simulink model "CMOS_Kernel_Memory_Sync"  (R2023b)
settings: Solver=VariableStepAuto  StartTime=0.0  StopTime=30000000  RelTol=1e-3
values from neighbouring files (symbols this model uses):
  AmountOfPixelsPerScanline = 400    [Kernel_Setup_Script.m]
  AmountOfRamBlocksScanlines = 5    [Kernel_Setup_Script.m]
  AmountOfRamBlocksScanlinesOffset = AmountOfRamBlocksScanlines - 1    (= 4)    [Kernel_Setup_Script.m]
  AmountOfScanlinePixels = 73700    [Kernel_Setup_Script.m]
  AmountOfScanlinePixelsOffset = AmountOfScanlinePixels - 1    (= 73699)    [Kernel_Setup_Script.m]
  AmountOfScanlines = 1100    [Kernel_Setup_Script.m]
  AmountOfScanlinesOffset = AmountOfScanlines - 1    (= 1099)    [Kernel_Setup_Script.m]
  AOPPK_Off = AmountOfPixelsPerScanline - 1    (= 399)    [Kernel_Setup_Script.m]
  AOPPS_Off = AmountOfPixelsPerScanline - 1    (= 399)    [Kernel_Setup_Script.m]
  FramePackOff_0 = FramePackOff_0 - ScanlineFifoCheck    [Kernel_Setup_Script.m]
  FramePackOff_1 = FramePackOff_1 - ScanlineFifoCheck    [Kernel_Setup_Script.m]
  FramePackOff_2 = FramePackOff_2 - ScanlineFifoCheck    [Kernel_Setup_Script.m]
  FramePackOff_3 = FramePackOff_3 - ScanlineFifoCheck    [Kernel_Setup_Script.m]
  FramePackOff_4 = FramePackOff_4 - ScanlineFifoCheck    [Kernel_Setup_Script.m]
  FramePackOff_5 = FramePackOff_5 - ScanlineFifoCheck    [Kernel_Setup_Script.m]
  KernelPackOff_0 = KernelPackOff_0 - KernelBitsPerRow    [Kernel_Setup_Script.m]
  KernelPackOff_1 = KernelPackOff_1 - KernelBitsPerRow    [Kernel_Setup_Script.m]
  KernelPackOff_2 = KernelPackOff_2 - KernelBitsPerRow    [Kernel_Setup_Script.m]
  KernelPackOff_3 = KernelPackOff_3 - KernelBitsPerRow    [Kernel_Setup_Script.m]
  Slice59DownTo48Top = (MsbOffset - (ScanlinePixelBitSizeController*1))    (= 59)    [Kernel_Setup_Script.m]
  Slice71DownTo60Top = (MsbOffset - (ScanlinePixelBitSizeController*0))    (= 71)    [Kernel_Setup_Script.m]
  TotalSectionsForFrames = AmountOfScanlines/AmountOfRamBlocksScanlines    (= 220)    [Kernel_Setup_Script.m]
  UltraRamRows = AmountOfPixelsPerScanline/ScanlineFifoCheck    [Kernel_Setup_Script.m]
  UltraRamRowsCeil = ceil(AmountOfPixelsPerScanline/ScanlineFifoCheck)    [Kernel_Setup_Script.m]
  UltraRamRowsKernel = AmountOfPixelsPerScanline/KernelBitsPerRow    (= 100)    [Kernel_Setup_Script.m]
  UltraRamRowsKernelCeil = ceil(AmountOfPixelsPerScanline/KernelBitsPerRow)    [Kernel_Setup_Script.m]
  UltraRamRowsMemorySectionOffset = UltraRamRowsCeil*AmountOfRamBlocksScanlines    [Kernel_Setup_Script.m]
  UltraRamRowsOffset = UltraRamRowsCeil - 1    [Kernel_Setup_Script.m]
undefined symbols (not defined in the file or in its folder): c, Down, sfvc784, Up, xck26
libraries: hdlBasic x4512, vmcUtilities x1
(part 2 of 39)

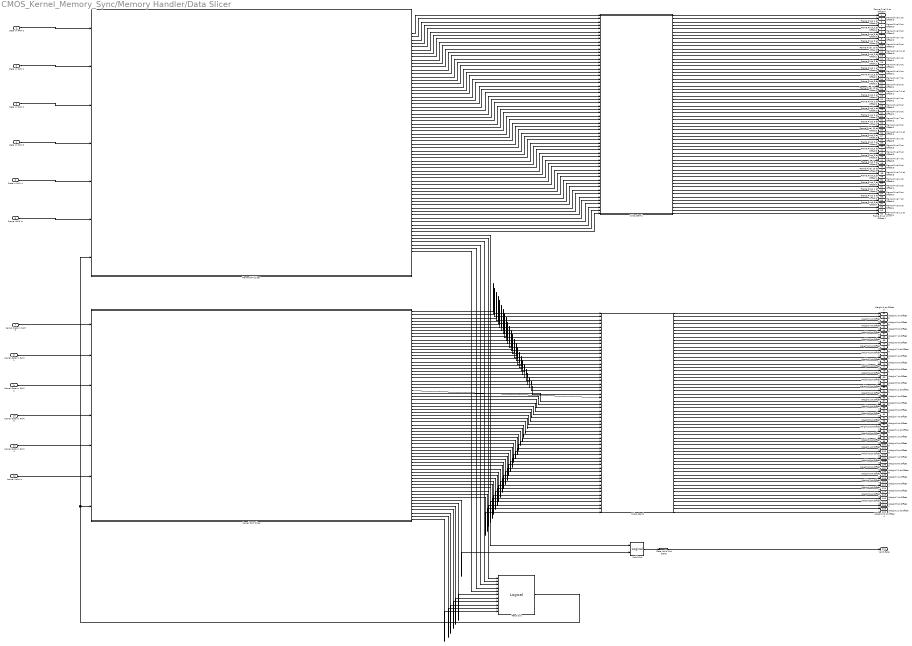
== system CMOS_Kernel_Memory_Sync/Memory Handler/Data Slicer ==
  Data In RAM 0 : Inport
  Data In RAM 1 : Inport  Port=2
  Data In RAM 2 : Inport  Port=3
  Data In RAM 3 : Inport  Port=4
  Data In RAM 4 : Inport  Port=5
  Frame Valid In : Inport  Port=6
  Kernel Data In RAM 0 : Inport  Port=7
  Kernel Data In RAM 1 : Inport  Port=8
  Kernel Data In RAM 2 : Inport  Port=9
  Kernel Data In RAM 3 : Inport  Port=10
  Kernel Data In RAM 4 : Inport  Port=11
  Kernel Valid In : Inport  Port=12
  Data Valid Out Delay : hdlBasic/Delay  rst=off  en=off  latency=1  reg_retiming=off  XmcBlockStatus=1  maskContainerNames=group1  block_type=delay  block_config=sysgen:Delay_config
  Frame RAM Slicer : Subsystem
      settings: RTWMemSecFuncInitTerm=Inherit fRAM model  RTWMemSecFuncExecute=Inherit fRAM model  RTWMemSecDataConstants=Inherit fRAM model  RTWMemSecDataInternal=Inherit fRAM model  RTWMemSecDataParameters=Inherit fRAM model
  Kernel RAM Slicer : Subsystem
      settings: RTWMemSecFuncInitTerm=Inherit fRAM model  RTWMemSecFuncExecute=Inherit fRAM model  RTWMemSecDataConstants=Inherit fRAM model  RTWMemSecDataInternal=Inherit fRAM model  RTWMemSecDataParameters=Inherit fRAM model
  Read Out : hdlBasic/Logical  logical_function=AND  inputs=11  en=off  latency=1  precision=User Defined  arith_type=Boolean  n_bits=1  bin_pt=0  align_bp=on  overflow=[]  quantization=[]  XmcBlockStatus=1  maskContainerNames=tabcontainer1  block_type=logical  block_config=sysgen:Logical_config
  Subsystem1 : Subsystem
      settings: RTWMemSecFuncInitTerm=Inherit fRAM model  RTWMemSecFuncExecute=Inherit fRAM model  RTWMemSecDataConstants=Inherit fRAM model  RTWMemSecDataInternal=Inherit fRAM model  RTWMemSecDataParameters=Inherit fRAM model
  Subsystem2 : Subsystem
      settings: RTWMemSecFuncInitTerm=Inherit fRAM model  RTWMemSecFuncExecute=Inherit fRAM model  RTWMemSecDataConstants=Inherit fRAM model  RTWMemSecDataInternal=Inherit fRAM model  RTWMemSecDataParameters=Inherit fRAM model
  Valid Out : hdlBasic/Logical  logical_function=AND  inputs=2  en=off  latency=1  precision=Full  arith_type=Unsigned  n_bits=16  bin_pt=0  align_bp=on  overflow=[]  quantization=[]  XmcBlockStatus=1  maskContainerNames=tabcontainer1  block_type=logical  block_config=sysgen:Logical_config
  Frame Pixel 0 at Offset 0 : Outport
  Frame Pixel 1 at Offset 0 : Outport  Port=2
  Frame Pixel 2 at Offset 0 : Outport  Port=3
  Frame Pixel 3 at Offset 0 : Outport  Port=4
  Frame Pixel 4 at Offset 0 : Outport  Port=5
  Frame Pixel 5 at Offset 0 : Outport  Port=6
  Frame Pixel 6 at Offset 0 : Outport  Port=7
  Frame Pixel 7 at Offset 0 : Outport  Port=8
  Frame Pixel 8 at Offset 0 : Outport  Port=9
  Frame Pixel 9 at Offset 0 : Outport  Port=10
  Frame Pixel 10 at Offset 0 : Outport  Port=11
  Frame Pixel 11 at Offset 0 : Outport  Port=12
  Frame Pixel 0 at Offset 1 : Outport  Port=13
  Frame Pixel 1 at Offset 1 : Outport  Port=14
  Frame Pixel 2 at Offset 1 : Outport  Port=15
  Frame Pixel 3 at Offset 1 : Outport  Port=16
  Frame Pixel 4 at Offset 1 : Outport  Port=17
  Frame Pixel 5 at Offset 1 : Outport  Port=18
  Frame Pixel 6 at Offset 1 : Outport  Port=19
  Frame Pixel 7 at Offset 1 : Outport  Port=20
  Frame Pixel 8 at Offset 1 : Outport  Port=21
  Frame Pixel 9 at Offset 1 : Outport  Port=22
  Frame Pixel 10 at Offset 1 : Outport  Port=23
  Frame Pixel 11 at Offset 1 : Outport  Port=24
  Frame Pixel 0 at Offset 2 : Outport  Port=25
  Frame Pixel 1 at Offset 2 : Outport  Port=26
  Frame Pixel 2 at Offset 2 : Outport  Port=27
  Frame Pixel 3 at Offset 2 : Outport  Port=28
  Frame Pixel 4 at Offset 2 : Outport  Port=29
  Frame Pixel 5 at Offset 2 : Outport  Port=30
  Frame Pixel 6 at Offset 2 : Outport  Port=31
  Frame Pixel 7 at Offset 2 : Outport  Port=32
  Frame Pixel 8 at Offset 2 : Outport  Port=33
  Frame Pixel 9 at Offset 2 : Outport  Port=34
  Frame Pixel 10 at Offset 2 : Outport  Port=35
  Frame Pixel 11 at Offset 2 : Outport  Port=36
  Frame Pixel 0 at Offset 3 : Outport  Port=37
  Frame Pixel 1 at Offset 3 : Outport  Port=38
  Frame Pixel 2 at Offset 3 : Outport  Port=39
  Frame Pixel 3 at Offset 3 : Outport  Port=40
  Frame Pixel 4 at Offset 3 : Outport  Port=41
  Frame Pixel 5 at Offset 3 : Outport  Port=42
  Frame Pixel 6 at Offset 3 : Outport  Port=43
  Frame Pixel 7 at Offset 3 : Outport  Port=44
  Frame Pixel 8 at Offset 3 : Outport  Port=45
  Frame Pixel 9 at Offset 3 : Outport  Port=46
  Frame Pixel 10 at Offset 3 : Outport  Port=47
  Frame Pixel 11 at Offset 3 : Outport  Port=48
  Frame Pixel 0 at Offset 4 : Outport  Port=49
  Frame Pixel 1 at Offset 4 : Outport  Port=50
  Frame Pixel 2 at Offset 4 : Outport  Port=51
  Frame Pixel 3 at Offset 4 : Outport  Port=52
  Frame Pixel 4 at Offset 4 : Outport  Port=53
  Frame Pixel 5 at Offset 4 : Outport  Port=54
  Frame Pixel 6 at Offset 4 : Outport  Port=55
  Frame Pixel 7 at Offset 4 : Outport  Port=56
  Frame Pixel 8 at Offset 4 : Outport  Port=57
  Frame Pixel 9 at Offset 4 : Outport  Port=58
  Frame Pixel 10 at Offset 4 : Outport  Port=59
  Frame Pixel 11 at Offset 4 : Outport  Port=60
  Weight 0 at Offset 0 : Outport  Port=61
  Weight 1 at Offset 0 : Outport  Port=62
  Weight 2 at Offset 0 : Outport  Port=63
  Weight 3 at Offset 0 : Outport  Port=64
  Weight 4 at Offset 0 : Outport  Port=65
  Weight 5 at Offset 0 : Outport  Port=66
  Weight 6 at Offset 0 : Outport  Port=67
  Weight 7 at Offset 0 : Outport  Port=68
  Weight 8 at Offset 0 : Outport  Port=69
  Weight 9 at Offset 0 : Outport  Port=70
  Weight 10 at Offset 0 : Outport  Port=71
  Weight 11 at Offset 0 : Outport  Port=72
  Weight 0 at Offset 1 : Outport  Port=73
  Weight 1 at Offset 1 : Outport  Port=74
  Weight 2 at Offset 1 : Outport  Port=75
  Weight 3 at Offset 1 : Outport  Port=76
  Weight 4 at Offset 1 : Outport  Port=77
  Weight 5 at Offset 1 : Outport  Port=78
  Weight 6 at Offset 1 : Outport  Port=79
  Weight 7 at Offset 1 : Outport  Port=80
  Weight 8 at Offset 1 : Outport  Port=81
  Weight 9 at Offset 1 : Outport  Port=82
  Weight 10 at Offset 1 : Outport  Port=83
  Weight 11 at Offset 1 : Outport  Port=84
  Weight 0 at Offset 2 : Outport  Port=85
  Weight 1 at Offset 2 : Outport  Port=86
  Weight 2 at Offset 2 : Outport  Port=87
  Weight 3 at Offset 2 : Outport  Port=88
  Weight 4 at Offset 2 : Outport  Port=89
  Weight 5 at Offset 2 : Outport  Port=90
  Weight 6 at Offset 2 : Outport  Port=91
  Weight 7 at Offset 2 : Outport  Port=92
  Weight 8 at Offset 2 : Outport  Port=93
  Weight 9 at Offset 2 : Outport  Port=94
  Weight 10 at Offset 2 : Outport  Port=95
  Weight 11 at Offset 2 : Outport  Port=96
  Weight 0 at Offset 3 : Outport  Port=97
  Weight 1 at Offset 3 : Outport  Port=98
  Weight 2 at Offset 3 : Outport  Port=99
  Weight 3 at Offset 3 : Outport  Port=100
  Weight 4 at Offset 3 : Outport  Port=101
  Weight 5 at Offset 3 : Outport  Port=102
  Weight 6 at Offset 3 : Outport  Port=103
  Weight 7 at Offset 3 : Outport  Port=104
  Weight 8 at Offset 3 : Outport  Port=105
  Weight 9 at Offset 3 : Outport  Port=106
  Weight 10 at Offset 3 : Outport  Port=107
  Weight 11 at Offset 3 : Outport  Port=108
  Weight 0 at Offset 4 : Outport  Port=109
  Weight 1 at Offset 4 : Outport  Port=110
  Weight 2 at Offset 4 : Outport  Port=111
  Weight 3 at Offset 4 : Outport  Port=112
  Weight 4 at Offset 4 : Outport  Port=113
  Weight 5 at Offset 4 : Outport  Port=114
  Weight 6 at Offset 4 : Outport  Port=115
  Weight 7 at Offset 4 : Outport  Port=116
  Weight 8 at Offset 4 : Outport  Port=117
  Weight 9 at Offset 4 : Outport  Port=118
  Weight 10 at Offset 4 : Outport  Port=119
  Weight 11 at Offset 4 : Outport  Port=120
  Valid Data : Outport  Port=121
  wires:
  Kernel RAM Slicer/61(Valid Out) -> Valid Out/2
  Frame RAM Slicer/61(Valid Out) -> Valid Out/1
  Frame RAM Slicer/1(Frame 12 Bit Bin Value 0 RAM 0) -> Subsystem1/1(Frame 12 Bit Bin Value 0)
  Frame RAM Slicer/2(Frame 12 Bit Bin Value 1 RAM 0) -> Subsystem1/2(Frame 12 Bit Bin Value 1)
  Frame RAM Slicer/3(Frame 12 Bit Bin Value 2 RAM 0) -> Subsystem1/3(Frame 12 Bit Bin Value 2)
  Frame RAM Slicer/4(Frame 12 Bit Bin Value 3 RAM 0) -> Subsystem1/4(Frame 12 Bit Bin Value 3)
  Frame RAM Slicer/5(Frame 12 Bit Bin Value 4 RAM 0) -> Subsystem1/5(Frame 12 Bit Bin Value 4)
  Frame RAM Slicer/6(Frame 12 Bit Bin Value 5 RAM 0) -> Subsystem1/6(Frame 12 Bit Bin Value 5)
  Frame RAM Slicer/7(Frame 12 Bit Bin Value 6 RAM 0) -> Subsystem1/7(Frame 12 Bit Bin Value 6)
  Frame RAM Slicer/8(Frame 12 Bit Bin Value 7 RAM 0) -> Subsystem1/8(Frame 12 Bit Bin Value 7)
  Frame RAM Slicer/9(Frame 12 Bit Bin Value 8 RAM 0) -> Subsystem1/9(Frame 12 Bit Bin Value 8)
  Frame RAM Slicer/10(Frame 12 Bit Bin Value 9 RAM 0) -> Subsystem1/10(Frame 12 Bit Bin Value 9)
  Frame RAM Slicer/11(Frame 12 Bit Bin Value 10 RAM 0) -> Subsystem1/11(Frame 12 Bit Bin Value 10)
  Frame RAM Slicer/12(Frame 12 Bit Bin Value 11 RAM 0) -> Subsystem1/12(Frame 12 Bit Bin Value 11)
  Frame RAM Slicer/13(Frame 12 Bit Bin Value 0 RAM 1) -> Subsystem1/13(Frame 12 Bit Bin Value 12)
  Frame RAM Slicer/14(Frame 12 Bit Bin Value 1 RAM 1) -> Subsystem1/14(Frame 12 Bit Bin Value 13)
  Frame RAM Slicer/15(Frame 12 Bit Bin Value 2 RAM 1) -> Subsystem1/15(Frame 12 Bit Bin Value 14)
  Frame RAM Slicer/16(Frame 12 Bit Bin Value 3 RAM 1) -> Subsystem1/16(Frame 12 Bit Bin Value 15)
  Frame RAM Slicer/17(Frame 12 Bit Bin Value 4 RAM 1) -> Subsystem1/17(Frame 12 Bit Bin Value 16)
  Frame RAM Slicer/18(Frame 12 Bit Bin Value 5 RAM 1) -> Subsystem1/18(Frame 12 Bit Bin Value 17)
  Frame RAM Slicer/19(Frame 12 Bit Bin Value 6 RAM 1) -> Subsystem1/19(Frame 12 Bit Bin Value 18)
  Frame RAM Slicer/20(Frame 12 Bit Bin Value 7 RAM 1) -> Subsystem1/20(Frame 12 Bit Bin Value 19)
  Frame RAM Slicer/21(Frame 12 Bit Bin Value 8 RAM 1) -> Subsystem1/21(Frame 12 Bit Bin Value 20)
  Frame RAM Slicer/22(Frame 12 Bit Bin Value 9 RAM 1) -> Subsystem1/22(Frame 12 Bit Bin Value 21)
  Frame RAM Slicer/23(Frame 12 Bit Bin Value 10 RAM 1) -> Subsystem1/23(Frame 12 Bit Bin Value 22)
  Frame RAM Slicer/24(Frame 12 Bit Bin Value 11 RAM 1) -> Subsystem1/24(Frame 12 Bit Bin Value 23)
  Frame RAM Slicer/25(Frame 12 Bit Bin Value 0 RAM 2) -> Subsystem1/25(Frame 12 Bit Bin Value 24)
  Frame RAM Slicer/26(Frame 12 Bit Bin Value 1 RAM 2) -> Subsystem1/26(Frame 12 Bit Bin Value 25)
  Frame RAM Slicer/27(Frame 12 Bit Bin Value 2 RAM 2) -> Subsystem1/27(Frame 12 Bit Bin Value 26)
  Frame RAM Slicer/28(Frame 12 Bit Bin Value 3 RAM 2) -> Subsystem1/28(Frame 12 Bit Bin Value 27)
  Frame RAM Slicer/29(Frame 12 Bit Bin Value 4 RAM 2) -> Subsystem1/29(Frame 12 Bit Bin Value 28)
  Frame RAM Slicer/30(Frame 12 Bit Bin Value 5 RAM 2) -> Subsystem1/30(Frame 12 Bit Bin Value 29)
  Frame RAM Slicer/31(Frame 12 Bit Bin Value 6 RAM 2) -> Subsystem1/31(Frame 12 Bit Bin Value 30)
  Frame RAM Slicer/32(Frame 12 Bit Bin Value 7 RAM 2) -> Subsystem1/32(Frame 12 Bit Bin Value 31)
  Frame RAM Slicer/33(Frame 12 Bit Bin Value 8 RAM 2) -> Subsystem1/33(Frame 12 Bit Bin Value 32)
  Frame RAM Slicer/34(Frame 12 Bit Bin Value 9 RAM 2) -> Subsystem1/34(Frame 12 Bit Bin Value 33)
  Frame RAM Slicer/35(Frame 12 Bit Bin Value 10 RAM 2) -> Subsystem1/35(Frame 12 Bit Bin Value 34)
  Frame RAM Slicer/36(Frame 12 Bit Bin Value 11 RAM 2) -> Subsystem1/36(Frame 12 Bit Bin Value 35)
  Frame RAM Slicer/42(Frame 12 Bit Bin Value 5 RAM 3) -> Subsystem1/42(Frame 12 Bit Bin Value 41)
  Frame RAM Slicer/37(Frame 12 Bit Bin Value 0 RAM 3) -> Subsystem1/37(Frame 12 Bit Bin Value 36)
  Frame RAM Slicer/54(Frame 12 Bit Bin Value 5 RAM 4) -> Subsystem1/54(Frame 12 Bit Bin Value 53)
  Frame RAM Slicer/57(Frame 12 Bit Bin Value 8 RAM 4) -> Subsystem1/57(Frame 12 Bit Bin Value 56)
  Frame RAM Slicer/47(Frame 12 Bit Bin Value 10 RAM 3) -> Subsystem1/47(Frame 12 Bit Bin Value 46)
  Frame RAM Slicer/53(Frame 12 Bit Bin Value 4 RAM 4) -> Subsystem1/53(Frame 12 Bit Bin Value 52)
  Frame RAM Slicer/44(Frame 12 Bit Bin Value 7 RAM 3) -> Subsystem1/44(Frame 12 Bit Bin Value 43)
  Frame RAM Slicer/51(Frame 12 Bit Bin Value 2 RAM 4) -> Subsystem1/51(Frame 12 Bit Bin Value 50)
  Frame RAM Slicer/58(Frame 12 Bit Bin Value 9 RAM 4) -> Subsystem1/58(Frame 12 Bit Bin Value 57)
  Frame RAM Slicer/56(Frame 12 Bit Bin Value 7 RAM 4) -> Subsystem1/56(Frame 12 Bit Bin Value 55)
  Frame RAM Slicer/52(Frame 12 Bit Bin Value 3 RAM 4) -> Subsystem1/52(Frame 12 Bit Bin Value 51)
  Frame RAM Slicer/43(Frame 12 Bit Bin Value 6 RAM 3) -> Subsystem1/43(Frame 12 Bit Bin Value 42)
  Frame RAM Slicer/49(Frame 12 Bit Bin Value 0 RAM 4) -> Subsystem1/49(Frame 12 Bit Bin Value 48)
  Frame RAM Slicer/40(Frame 12 Bit Bin Value 3 RAM 3) -> Subsystem1/40(Frame 12 Bit Bin Value 39)
  Frame RAM Slicer/46(Frame 12 Bit Bin Value 9 RAM 3) -> Subsystem1/46(Frame 12 Bit Bin Value 45)
  Frame RAM Slicer/55(Frame 12 Bit Bin Value 6 RAM 4) -> Subsystem1/55(Frame 12 Bit Bin Value 54)
  Frame RAM Slicer/39(Frame 12 Bit Bin Value 2 RAM 3) -> Subsystem1/39(Frame 12 Bit Bin Value 38)
  Frame RAM Slicer/45(Frame 12 Bit Bin Value 8 RAM 3) -> Subsystem1/45(Frame 12 Bit Bin Value 44)
  Frame RAM Slicer/60(Frame 12 Bit Bin Value 11 RAM 4) -> Subsystem1/60(Frame 12 Bit Bin Value 59)
  Frame RAM Slicer/59(Frame 12 Bit Bin Value 10 RAM 4) -> Subsystem1/59(Frame 12 Bit Bin Value 58)
  Frame RAM Slicer/41(Frame 12 Bit Bin Value 4 RAM 3) -> Subsystem1/41(Frame 12 Bit Bin Value 40)
  Frame RAM Slicer/50(Frame 12 Bit Bin Value 1 RAM 4) -> Subsystem1/50(Frame 12 Bit Bin Value 49)
  Frame RAM Slicer/48(Frame 12 Bit Bin Value 11 RAM 3) -> Subsystem1/48(Frame 12 Bit Bin Value 47)
  Frame RAM Slicer/38(Frame 12 Bit Bin Value 1 RAM 3) -> Subsystem1/38(Frame 12 Bit Bin Value 37)
  Data In RAM 0/1 -> Frame RAM Slicer/1(Data In RAM 0)
  Data In RAM 2/1 -> Frame RAM Slicer/3(Data In RAM 2)
  Data In RAM 3/1 -> Frame RAM Slicer/4(Data In RAM 3)
  Data In RAM 4/1 -> Frame RAM Slicer/5(Data In RAM 4)
  Frame Valid In/1 -> Frame RAM Slicer/6(Valid In)
  Kernel Data In RAM 0/1 -> Kernel RAM Slicer/1(Kernel Data In RAM 0)
  Kernel Data In RAM 1/1 -> Kernel RAM Slicer/2(Kernel Data In RAM 1)
  Kernel Data In RAM 2/1 -> Kernel RAM Slicer/3(Kernel Data In RAM 2)
  Kernel Data In RAM 3/1 -> Kernel RAM Slicer/4(Kernel Data In RAM 3)
  Kernel Data In RAM 4/1 -> Kernel RAM Slicer/5(Kernel Data In RAM 4)
  Kernel Valid In/1 -> Kernel RAM Slicer/6(Valid In)
  Data In RAM 1/1 -> Frame RAM Slicer/2(Data In RAM 1)
  Valid Out/1 -> Data Valid Out Delay/1
  Kernel RAM Slicer/1(Kernel 18 Bit Value 0 RAM 0) -> Subsystem2/1(Kernel 18 Bit Bin Value 0)
  Kernel RAM Slicer/2(Kernel 18 Bit Value 1 RAM 0) -> Subsystem2/2(Kernel 18 Bit Bin Value 1)
  Kernel RAM Slicer/3(Kernel 18 Bit Value 2 RAM 0) -> Subsystem2/3(Kernel 18 Bit Bin Value 2)
  Kernel RAM Slicer/4(Kernel 18 Bit Value 3 RAM 0) -> Subsystem2/4(Kernel 18 Bit Bin Value 3)
  Kernel RAM Slicer/5(Kernel 18 Bit Value 4 RAM 0) -> Subsystem2/5(Kernel 18 Bit Bin Value 4)
  Kernel RAM Slicer/6(Kernel 18 Bit Value 5 RAM 0) -> Subsystem2/6(Kernel 18 Bit Bin Value 5)
  Kernel RAM Slicer/7(Kernel 18 Bit Value 6 RAM 0) -> Subsystem2/7(Kernel 18 Bit Bin Value 6)
  Kernel RAM Slicer/8(Kernel 18 Bit Value 7 RAM 0) -> Subsystem2/8(Kernel 18 Bit Bin Value 7)
  Kernel RAM Slicer/9(Kernel 18 Bit Value 8 RAM 0) -> Subsystem2/9(Kernel 18 Bit Bin Value 8)
  Kernel RAM Slicer/10(Kernel 18 Bit Value 9 RAM 0) -> Subsystem2/10(Kernel 18 Bit Bin Value 9)
  Kernel RAM Slicer/11(Kernel 18 Bit Value 10 RAM 0) -> Subsystem2/11(Kernel 18 Bit Bin Value 10)
  Kernel RAM Slicer/12(Kernel 18 Bit Value 11 RAM 0) -> Subsystem2/12(Kernel 18 Bit Bin Value 11)
  Kernel RAM Slicer/13(Kernel 18 Bit Value 0 RAM 1) -> Subsystem2/13(Kernel 18 Bit Bin Value 12)
  Kernel RAM Slicer/14(Kernel 18 Bit Value 1 RAM 1) -> Subsystem2/14(Kernel 18 Bit Bin Value 13)
  Kernel RAM Slicer/15(Kernel 18 Bit Value 2 RAM 1) -> Subsystem2/15(Kernel 18 Bit Bin Value 14)
  Kernel RAM Slicer/16(Kernel 18 Bit Value 3 RAM 1) -> Subsystem2/16(Kernel 18 Bit Bin Value 15)
  Kernel RAM Slicer/17(Kernel 18 Bit Value 4 RAM 1) -> Subsystem2/17(Kernel 18 Bit Bin Value 16)
  Kernel RAM Slicer/18(Kernel 18 Bit Value 5 RAM 1) -> Subsystem2/18(Kernel 18 Bit Bin Value 17)
  Kernel RAM Slicer/19(Kernel 18 Bit Value 6 RAM 1) -> Subsystem2/19(Kernel 18 Bit Bin Value 18)
  Kernel RAM Slicer/20(Kernel 18 Bit Value 7 RAM 1) -> Subsystem2/20(Kernel 18 Bit Bin Value 19)
  Kernel RAM Slicer/21(Kernel 18 Bit Value 8 RAM 1) -> Subsystem2/21(Kernel 18 Bit Bin Value 20)
  Kernel RAM Slicer/22(Kernel 18 Bit Value 9 RAM 1) -> Subsystem2/22(Kernel 18 Bit Bin Value 21)
  Kernel RAM Slicer/23(Kernel 18 Bit Value 10 RAM 1) -> Subsystem2/23(Kernel 18 Bit Bin Value 22)
  Kernel RAM Slicer/24(Kernel 18 Bit Value 11 RAM 1) -> Subsystem2/24(Kernel 18 Bit Bin Value 23)
  Kernel RAM Slicer/25(Kernel 18 Bit Value 0 RAM 2) -> Subsystem2/25(Kernel 18 Bit Bin Value 24)
  Kernel RAM Slicer/26(Kernel 18 Bit Value 1 RAM 2) -> Subsystem2/26(Kernel 18 Bit Bin Value 25)
  Kernel RAM Slicer/27(Kernel 18 Bit Value 2 RAM 2) -> Subsystem2/27(Kernel 18 Bit Bin Value 26)
  Kernel RAM Slicer/28(Kernel 18 Bit Value 3 RAM 2) -> Subsystem2/28(Kernel 18 Bit Bin Value 27)
  Kernel RAM Slicer/29(Kernel 18 Bit Value 4 RAM 2) -> Subsystem2/29(Kernel 18 Bit Bin Value 28)
  Kernel RAM Slicer/30(Kernel 18 Bit Value 5 RAM 2) -> Subsystem2/30(Kernel 18 Bit Bin Value 29)
  Kernel RAM Slicer/31(Kernel 18 Bit Value 6 RAM 2) -> Subsystem2/31(Kernel 18 Bit Bin Value 30)
  Kernel RAM Slicer/32(Kernel 18 Bit Value 7 RAM 2) -> Subsystem2/32(Kernel 18 Bit Bin Value 31)
  Kernel RAM Slicer/33(Kernel 18 Bit Value 8 RAM 2) -> Subsystem2/33(Kernel 18 Bit Bin Value 32)
  Kernel RAM Slicer/34(Kernel 18 Bit Value 9 RAM 2) -> Subsystem2/34(Kernel 18 Bit Bin Value 33)
  Kernel RAM Slicer/35(Kernel 18 Bit Value 10 RAM 2) -> Subsystem2/35(Kernel 18 Bit Bin Value 34)
  Kernel RAM Slicer/36(Kernel 18 Bit Value 11 RAM 2) -> Subsystem2/36(Kernel 18 Bit Bin Value 35)
  Kernel RAM Slicer/37(Kernel 18 Bit Value 0 RAM 3) -> Subsystem2/37(Kernel 18 Bit Bin Value 36)
  Kernel RAM Slicer/38(Kernel 18 Bit Value 1 RAM 3) -> Subsystem2/38(Kernel 18 Bit Bin Value 37)
  Kernel RAM Slicer/39(Kernel 18 Bit Value 2 RAM 3) -> Subsystem2/39(Kernel 18 Bit Bin Value 38)
  Kernel RAM Slicer/40(Kernel 18 Bit Value 3 RAM 3) -> Subsystem2/40(Kernel 18 Bit Bin Value 39)
  Kernel RAM Slicer/41(Kernel 18 Bit Value 4 RAM 3) -> Subsystem2/41(Kernel 18 Bit Bin Value 40)
  Kernel RAM Slicer/42(Kernel 18 Bit Value 5 RAM 3) -> Subsystem2/42(Kernel 18 Bit Bin Value 41)
  Kernel RAM Slicer/43(Kernel 18 Bit Value 6 RAM 3) -> Subsystem2/43(Kernel 18 Bit Bin Value 42)
  Kernel RAM Slicer/44(Kernel 18 Bit Value 7 RAM 3) -> Subsystem2/44(Kernel 18 Bit Bin Value 43)
  Kernel RAM Slicer/45(Kernel 18 Bit Value 8 RAM 3) -> Subsystem2/45(Kernel 18 Bit Bin Value 44)
  Kernel RAM Slicer/46(Kernel 18 Bit Value 9 RAM 3) -> Subsystem2/46(Kernel 18 Bit Bin Value 45)
  Kernel RAM Slicer/47(Kernel 18 Bit Value 10 RAM 3) -> Subsystem2/47(Kernel 18 Bit Bin Value 46)
  Kernel RAM Slicer/48(Kernel 18 Bit Value 11 RAM 3) -> Subsystem2/48(Kernel 18 Bit Bin Value 47)
  Kernel RAM Slicer/49(Kernel 18 Bit Value 0 RAM 4) -> Subsystem2/49(Kernel 18 Bit Bin Value 48)
  Kernel RAM Slicer/50(Kernel 18 Bit Value 1 RAM 4) -> Subsystem2/50(Kernel 18 Bit Bin Value 49)
  Kernel RAM Slicer/51(Kernel 18 Bit Value 2 RAM 4) -> Subsystem2/51(Kernel 18 Bit Bin Value 50)
  Kernel RAM Slicer/52(Kernel 18 Bit Value 3 RAM 4) -> Subsystem2/52(Kernel 18 Bit Bin Value 51)
  Kernel RAM Slicer/53(Kernel 18 Bit Value 4 RAM 4) -> Subsystem2/53(Kernel 18 Bit Bin Value 52)
  Kernel RAM Slicer/54(Kernel 18 Bit Value 5 RAM 4) -> Subsystem2/54(Kernel 18 Bit Bin Value 53)
  Kernel RAM Slicer/55(Kernel 18 Bit Value 6 RAM 4) -> Subsystem2/55(Kernel 18 Bit Bin Value 54)
  Kernel RAM Slicer/56(Kernel 18 Bit Value 7 RAM 4) -> Subsystem2/56(Kernel 18 Bit Bin Value 55)
  Kernel RAM Slicer/57(Kernel 18 Bit Value 8 RAM 4) -> Subsystem2/57(Kernel 18 Bit Bin Value 56)
  Kernel RAM Slicer/58(Kernel 18 Bit Value 9 RAM 4) -> Subsystem2/58(Kernel 18 Bit Bin Value 57)
  Kernel RAM Slicer/59(Kernel 18 Bit Value 10 RAM 4) -> Subsystem2/59(Kernel 18 Bit Bin Value 58)
  Kernel RAM Slicer/60(Kernel 18 Bit Value 11 RAM 4) -> Subsystem2/60(Kernel 18 Bit Bin Value 59)
  Subsystem1/1(Frame 12 Bit Value 0) -> Frame Pixel 0 at Offset 0/1
  Subsystem1/2(Frame 12 Bit Value 1) -> Frame Pixel 1 at Offset 0/1
  Subsystem1/3(Frame 12 Bit Value 2) -> Frame Pixel 2 at Offset 0/1
  Subsystem1/4(Frame 12 Bit Value 3) -> Frame Pixel 3 at Offset 0/1
  Subsystem1/7(Frame 12 Bit Value 6) -> Frame Pixel 6 at Offset 0/1
  Subsystem1/8(Frame 12 Bit Value 7) -> Frame Pixel 7 at Offset 0/1
  Subsystem1/5(Frame 12 Bit Value 4) -> Frame Pixel 4 at Offset 0/1
  Subsystem1/6(Frame 12 Bit Value 5) -> Frame Pixel 5 at Offset 0/1
  Subsystem1/11(Frame 12 Bit Value 10) -> Frame Pixel 10 at Offset 0/1
  Subsystem1/9(Frame 12 Bit Value 8) -> Frame Pixel 8 at Offset 0/1
  Subsystem1/10(Frame 12 Bit Value 9) -> Frame Pixel 9 at Offset 0/1
  Subsystem1/12(Frame 12 Bit Value 11) -> Frame Pixel 11 at Offset 0/1
  Subsystem1/24(Frame 12 Bit Value 23) -> Frame Pixel 11 at Offset 1/1
  Subsystem1/23(Frame 12 Bit Value 22) -> Frame Pixel 10 at Offset 1/1
  Subsystem1/22(Frame 12 Bit Value 21) -> Frame Pixel 9 at Offset 1/1
  Subsystem1/21(Frame 12 Bit Value 20) -> Frame Pixel 8 at Offset 1/1
  Subsystem1/15(Frame 12 Bit Value 14) -> Frame Pixel 2 at Offset 1/1
  Subsystem1/17(Frame 12 Bit Value 16) -> Frame Pixel 4 at Offset 1/1
  Subsystem1/13(Frame 12 Bit Value 12) -> Frame Pixel 0 at Offset 1/1
  Subsystem1/14(Frame 12 Bit Value 13) -> Frame Pixel 1 at Offset 1/1
  Subsystem1/18(Frame 12 Bit Value 17) -> Frame Pixel 5 at Offset 1/1
  Subsystem1/19(Frame 12 Bit Value 18) -> Frame Pixel 6 at Offset 1/1
  Subsystem1/16(Frame 12 Bit Value 15) -> Frame Pixel 3 at Offset 1/1
  Subsystem1/20(Frame 12 Bit Value 19) -> Frame Pixel 7 at Offset 1/1
  Subsystem1/36(Frame 12 Bit Value 35) -> Frame Pixel 11 at Offset 2/1
  Subsystem1/35(Frame 12 Bit Value 34) -> Frame Pixel 10 at Offset 2/1
  Subsystem1/34(Frame 12 Bit Value 33) -> Frame Pixel 9 at Offset 2/1
  Subsystem1/33(Frame 12 Bit Value 32) -> Frame Pixel 8 at Offset 2/1
  Subsystem1/27(Frame 12 Bit Value 26) -> Frame Pixel 2 at Offset 2/1
  Subsystem1/29(Frame 12 Bit Value 28) -> Frame Pixel 4 at Offset 2/1
  Subsystem1/25(Frame 12 Bit Value 24) -> Frame Pixel 0 at Offset 2/1
  Subsystem1/26(Frame 12 Bit Value 25) -> Frame Pixel 1 at Offset 2/1
  Subsystem1/30(Frame 12 Bit Value 29) -> Frame Pixel 5 at Offset 2/1
  Subsystem1/31(Frame 12 Bit Value 30) -> Frame Pixel 6 at Offset 2/1
  Subsystem1/28(Frame 12 Bit Value 27) -> Frame Pixel 3 at Offset 2/1
  Subsystem1/32(Frame 12 Bit Value 31) -> Frame Pixel 7 at Offset 2/1
  Subsystem1/48(Frame 12 Bit Value 47) -> Frame Pixel 11 at Offset 3/1
  Subsystem1/47(Frame 12 Bit Value 46) -> Frame Pixel 10 at Offset 3/1
  Subsystem1/46(Frame 12 Bit Value 45) -> Frame Pixel 9 at Offset 3/1
  Subsystem1/45(Frame 12 Bit Value 44) -> Frame Pixel 8 at Offset 3/1
  Subsystem1/39(Frame 12 Bit Value 38) -> Frame Pixel 2 at Offset 3/1
  Subsystem1/41(Frame 12 Bit Value 40) -> Frame Pixel 4 at Offset 3/1
  Subsystem1/37(Frame 12 Bit Value 36) -> Frame Pixel 0 at Offset 3/1
  Subsystem1/38(Frame 12 Bit Value 37) -> Frame Pixel 1 at Offset 3/1
  Subsystem1/42(Frame 12 Bit Value 41) -> Frame Pixel 5 at Offset 3/1
  Subsystem1/43(Frame 12 Bit Value 42) -> Frame Pixel 6 at Offset 3/1
  Subsystem1/40(Frame 12 Bit Value 39) -> Frame Pixel 3 at Offset 3/1
  Subsystem1/44(Frame 12 Bit Value 43) -> Frame Pixel 7 at Offset 3/1
  Subsystem1/60(Frame 12 Bit Value 59) -> Frame Pixel 11 at Offset 4/1
  Subsystem1/59(Frame 12 Bit Value 58) -> Frame Pixel 10 at Offset 4/1
  Subsystem1/58(Frame 12 Bit Value 57) -> Frame Pixel 9 at Offset 4/1
  Subsystem1/57(Frame 12 Bit Value 56) -> Frame Pixel 8 at Offset 4/1
  Subsystem1/51(Frame 12 Bit Value 50) -> Frame Pixel 2 at Offset 4/1
  Subsystem1/53(Frame 12 Bit Value 52) -> Frame Pixel 4 at Offset 4/1
  Subsystem1/49(Frame 12 Bit Value 48) -> Frame Pixel 0 at Offset 4/1
  Subsystem1/50(Frame 12 Bit Value 49) -> Frame Pixel 1 at Offset 4/1
  Subsystem1/54(Frame 12 Bit Value 53) -> Frame Pixel 5 at Offset 4/1
  Subsystem1/55(Frame 12 Bit Value 54) -> Frame Pixel 6 at Offset 4/1
  Subsystem1/52(Frame 12 Bit Value 51) -> Frame Pixel 3 at Offset 4/1
  Subsystem1/56(Frame 12 Bit Value 55) -> Frame Pixel 7 at Offset 4/1
  Subsystem2/12(Kernel 18 Bit Value 11) -> Weight 11 at Offset 0/1
  Subsystem2/11(Kernel 18 Bit Value 10) -> Weight 10 at Offset 0/1
  Subsystem2/10(Kernel 18 Bit Value 9) -> Weight 9 at Offset 0/1
  Subsystem2/9(Kernel 18 Bit Value 8) -> Weight 8 at Offset 0/1
  Subsystem2/3(Kernel 18 Bit Value 2) -> Weight 2 at Offset 0/1
  Subsystem2/5(Kernel 18 Bit Value 4) -> Weight 4 at Offset 0/1
  Subsystem2/1(Kernel 18 Bit Value 0) -> Weight 0 at Offset 0/1
  Subsystem2/2(Kernel 18 Bit Value 1) -> Weight 1 at Offset 0/1
  Subsystem2/6(Kernel 18 Bit Value 5) -> Weight 5 at Offset 0/1
  Subsystem2/7(Kernel 18 Bit Value 6) -> Weight 6 at Offset 0/1
  Subsystem2/4(Kernel 18 Bit Value 3) -> Weight 3 at Offset 0/1
  Subsystem2/8(Kernel 18 Bit Value 7) -> Weight 7 at Offset 0/1
  Subsystem2/24(Kernel 18 Bit Value 23) -> Weight 11 at Offset 1/1
  Subsystem2/18(Kernel 18 Bit Value 17) -> Weight 5 at Offset 1/1
  Subsystem2/21(Kernel 18 Bit Value 20) -> Weight 8 at Offset 1/1
  Subsystem2/20(Kernel 18 Bit Value 19) -> Weight 7 at Offset 1/1
  Subsystem2/23(Kernel 18 Bit Value 22) -> Weight 10 at Offset 1/1
  Subsystem2/13(Kernel 18 Bit Value 12) -> Weight 0 at Offset 1/1
  Subsystem2/19(Kernel 18 Bit Value 18) -> Weight 6 at Offset 1/1
  Subsystem2/22(Kernel 18 Bit Value 21) -> Weight 9 at Offset 1/1
  Subsystem2/16(Kernel 18 Bit Value 15) -> Weight 3 at Offset 1/1
  Subsystem2/15(Kernel 18 Bit Value 14) -> Weight 2 at Offset 1/1
  Subsystem2/14(Kernel 18 Bit Value 13) -> Weight 1 at Offset 1/1
  Subsystem2/17(Kernel 18 Bit Value 16) -> Weight 4 at Offset 1/1
  Subsystem2/36(Kernel 18 Bit Value 35) -> Weight 11 at Offset 2/1
  Subsystem2/30(Kernel 18 Bit Value 29) -> Weight 5 at Offset 2/1
  Subsystem2/33(Kernel 18 Bit Value 32) -> Weight 8 at Offset 2/1
  Subsystem2/32(Kernel 18 Bit Value 31) -> Weight 7 at Offset 2/1
  Subsystem2/35(Kernel 18 Bit Value 34) -> Weight 10 at Offset 2/1
  Subsystem2/25(Kernel 18 Bit Value 24) -> Weight 0 at Offset 2/1
  Subsystem2/31(Kernel 18 Bit Value 30) -> Weight 6 at Offset 2/1
  Subsystem2/34(Kernel 18 Bit Value 33) -> Weight 9 at Offset 2/1
  Subsystem2/28(Kernel 18 Bit Value 27) -> Weight 3 at Offset 2/1
  Subsystem2/27(Kernel 18 Bit Value 26) -> Weight 2 at Offset 2/1
  Subsystem2/26(Kernel 18 Bit Value 25) -> Weight 1 at Offset 2/1
  Subsystem2/29(Kernel 18 Bit Value 28) -> Weight 4 at Offset 2/1
  Subsystem2/48(Kernel 18 Bit Value 47) -> Weight 11 at Offset 3/1
  Subsystem2/42(Kernel 18 Bit Value 41) -> Weight 5 at Offset 3/1
  Subsystem2/45(Kernel 18 Bit Value 44) -> Weight 8 at Offset 3/1
  Subsystem2/44(Kernel 18 Bit Value 43) -> Weight 7 at Offset 3/1
  Subsystem2/47(Kernel 18 Bit Value 46) -> Weight 10 at Offset 3/1
  Subsystem2/37(Kernel 18 Bit Value 36) -> Weight 0 at Offset 3/1
  Subsystem2/43(Kernel 18 Bit Value 42) -> Weight 6 at Offset 3/1
  Subsystem2/46(Kernel 18 Bit Value 45) -> Weight 9 at Offset 3/1
  Subsystem2/40(Kernel 18 Bit Value 39) -> Weight 3 at Offset 3/1
  Subsystem2/39(Kernel 18 Bit Value 38) -> Weight 2 at Offset 3/1
  Subsystem2/38(Kernel 18 Bit Value 37) -> Weight 1 at Offset 3/1
  Subsystem2/41(Kernel 18 Bit Value 40) -> Weight 4 at Offset 3/1
  Subsystem2/60(Kernel 18 Bit Value 59) -> Weight 11 at Offset 4/1
  Subsystem2/54(Kernel 18 Bit Value 53) -> Weight 5 at Offset 4/1
  Subsystem2/57(Kernel 18 Bit Value 56) -> Weight 8 at Offset 4/1
  Subsystem2/56(Kernel 18 Bit Value 55) -> Weight 7 at Offset 4/1
  Subsystem2/59(Kernel 18 Bit Value 58) -> Weight 10 at Offset 4/1
  Subsystem2/49(Kernel 18 Bit Value 48) -> Weight 0 at Offset 4/1
  Subsystem2/55(Kernel 18 Bit Value 54) -> Weight 6 at Offset 4/1
  Subsystem2/58(Kernel 18 Bit Value 57) -> Weight 9 at Offset 4/1
  Subsystem2/52(Kernel 18 Bit Value 51) -> Weight 3 at Offset 4/1
  Subsystem2/51(Kernel 18 Bit Value 50) -> Weight 2 at Offset 4/1
  Subsystem2/50(Kernel 18 Bit Value 49) -> Weight 1 at Offset 4/1
  Subsystem2/53(Kernel 18 Bit Value 52) -> Weight 4 at Offset 4/1
  Data Valid Out Delay/1 -> Valid Data/1
  Frame RAM Slicer/62(Wrote to Last FIFO RAM 0) -> Read Out/1
  Frame RAM Slicer/63(Wrote to Last FIFO RAM 1) -> Read Out/2
  Frame RAM Slicer/64(Wrote to Last FIFO RAM 2) -> Read Out/3
  Frame RAM Slicer/65(Wrote to Last FIFO RAM 3) -> Read Out/4
  Frame RAM Slicer/66(Wrote to Last FIFO RAM 4) -> Read Out/5
  Kernel RAM Slicer/62(Wrote to Last FIFO RAM 0) -> Read Out/6
  Kernel RAM Slicer/63(Wrote to Last FIFO RAM 1) -> Read Out/7
  Kernel RAM Slicer/64(Wrote to Last FIFO RAM 2) -> Read Out/8
  Kernel RAM Slicer/65(Wrote to Last FIFO RAM 3) -> Read Out/9
  Kernel RAM Slicer/66(Wrote to Last FIFO RAM 4) -> Read Out/10
  Read Out/1 -> Kernel RAM Slicer/7(Read Enable), Frame RAM Slicer/7(Read Enable)
  Kernel RAM Slicer/67(Wrote to last FIFO Trigger) -> Read Out/11
